simulink model "Simulink_test"  (R2015b)
settings: Solver=VariableStepAuto  StartTime=0.0  StopTime=20  RelTol=1e-3
libraries: simulink x3
settings Model: Creator=Ecslogon2  LastModifiedBy=Ecslogon2

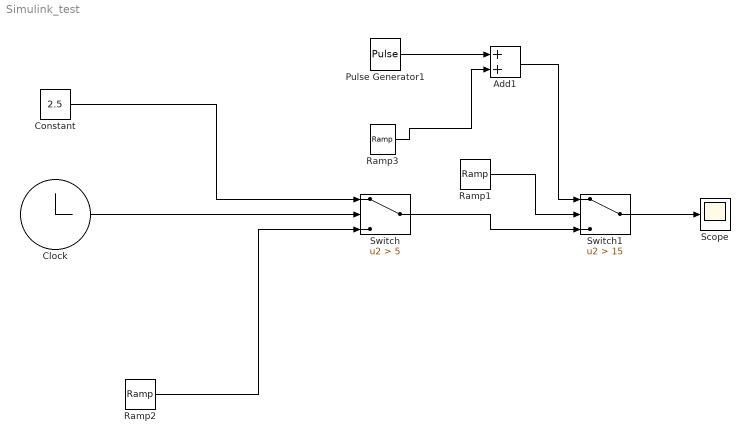
== system Simulink_test ==
  Add1 : Sum
  Clock : Clock
      settings: Decimation=20
  Constant : Constant  Value=2.5
  Pulse Generator1 : DiscretePulseGenerator  PulseType=Time based  Amplitude=.5  PulseWidth=5
  Ramp1 : simulink/Sources/Ramp  slope=1  start=0  X0=0
  Ramp2 : simulink/Sources/Ramp  slope=.5  start=0  X0=0
  Ramp3 : simulink/Sources/Ramp  slope=-.5  start=15  X0=2.5
  Scope : Scope
  Switch : Switch  Criteria=u2 > Threshold  Threshold=5
  Switch1 : Switch  Criteria=u2 > Threshold  Threshold=15
  wires:
  Clock/1 -> Switch/2
  Switch/1 -> Switch1/3
  Ramp1/1 -> Switch1/2
  Switch1/1 -> Scope/1
  Ramp3/1 -> Add1/2
  Pulse Generator1/1 -> Add1/1
  Add1/1 -> Switch1/1
  Constant/1 -> Switch/1
  Ramp2/1 -> Switch/3
